simulink model "CallbackLianxi"  (Simulink 9.1)
settings: Solver=VariableStepAuto  StartTime=0.0  StopTime=10.0  RelTol=1e-3
PreLoadFcn:
  | clear
  | AAA=rand;
  | flag=0;
StartFcn:
  | warndlg('仿真开始了！','')
settings Model: Creator=McQueen_Zero  LastModifiedBy=McQueen_Zero
settings DataIOCC: SaveFormat=Dataset
settings OptimizationCC: LifeSpan=auto
settings DebuggingCC: UnderspecifiedInitializationDetection=Simplified  MergeDetectMultiDrivingBlocksExec=error  SFUnexpectedBacktrackingDiag=error  SFNoUnconditionalDefaultTransitionDiag=error  SFExecutionAtInitializationDiag=warning
settings HardwareCC: ProdBitPerPointer=64  ProdBitPerSizeT=64  ProdBitPerPtrDiffT=64  ProdLargestAtomicFloat=Float  ProdIntDivRoundTo=Zero  ProdEndianess=LittleEndian  ProdWordSize=64  ProdHWDeviceType=Intel->x86-64 (Windows64)
settings ModelReferenceCC: PropagateSignalLabelsOutOfModel=on
settings CodeAppCC: StateflowObjectComments=off
settings GRTTargetCC: TargetLangStandard=C99 (ISO)  CombineOutputUpdateFcns=on  GRTInterface=off
settings ConfigComp: CovMetricSettings=dwe  CovHtmlReporting=off  CovSaveCumulativeToWorkspaceVar=off  CovSaveSingleToWorkspaceVar=off  CovExternalEMLEnable=on

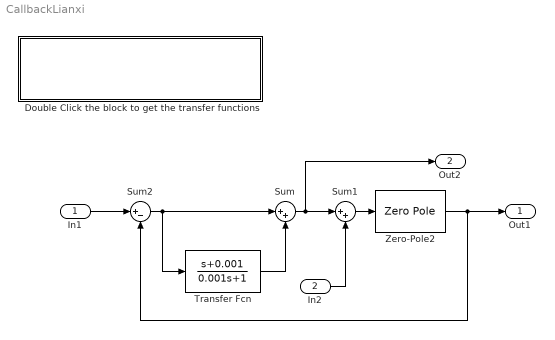
== system CallbackLianxi ==
  In1 : Inport
  In2 : Inport  Port=2
  Double Click the block to get the transfer functions : Subsystem  Description=text('Double Click to get the transfer function')
      settings: OpenFcn=|
      | clc;
      | clear;
      | [A,B,C,D]=linmod('CallbackLianxi');
      | G=ss(A,B,C,D);
      | G=tf(G);
      | disp('所求的传递函数如下所示：')
      | minreal(zpk(G))
  Sum : Sum  Inputs=|++
  Sum1 : Sum  Inputs=|++
  Sum2 : Sum  Inputs=|+-  SaturateOnIntegerOverflow=on
  Transfer Fcn : TransferFcn  Numerator=[1 0.001]  Denominator=[0.001 1]
      settings: MoveFcn=|
      | if flag==0
      | warndlg('别动我，烦着呢！','')
      | flag=1;
      | else
      | warndlg('再动我一下试试？！','')
      | flag=0;
      | end
  Zero-Pole2 : ZeroPole  Zeros=[]  Poles=[ -0.5]
  Out1 : Outport
  Out2 : Outport  Port=2
  wires:
  Sum1/1 -> Zero-Pole2/1
  Transfer Fcn/1 -> Sum/2
  In1/1 -> Sum2/1
  In2/1 -> Sum1/2
  Sum/1 -> Out2/1, Sum1/1
  Sum2/1 -> Sum/1, Transfer Fcn/1
  Zero-Pole2/1 -> Sum2/2, Out1/1

== system CallbackLianxi/Double Click the block to get the transfer functions ==
